simulink model "linear_system_full_state_obs"  (R2021b)
settings: Solver=VariableStepAuto  StartTime=0.0  StopTime=10.0  RelTol=1e-8
undefined symbols (not defined in the file or in its folder): A, B, K
libraries: simulink x2
settings Model: Creator=viking  LastModifiedBy=viking
settings DebuggingCC: UnconnectedInputMsg=none  UnconnectedOutputMsg=none  UnconnectedLineMsg=none
settings ModelReferenceCC: EnableRefExpFcnMdlSchedulingChecks=off
settings RTWCC: DLArmComputeVersion=20.02.1

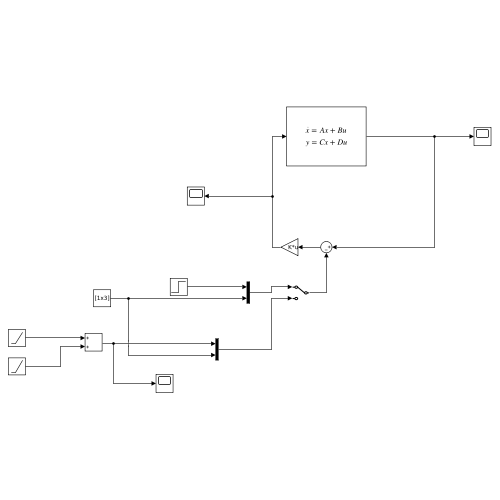
[thumbnail: Simulink's stored preview of the top-level diagram]
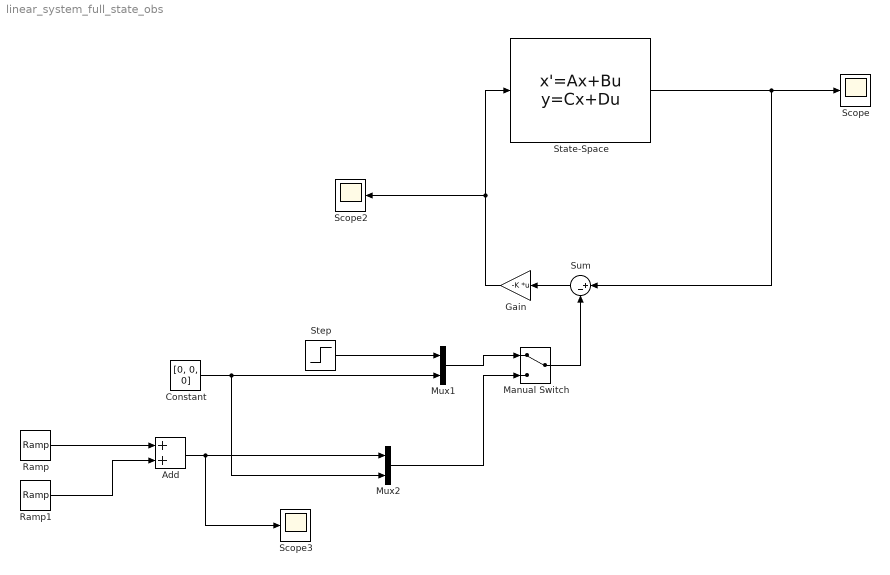
== system linear_system_full_state_obs ==
  Add : Sum
  Constant : Constant  Value=[0, 0, 0]
  Gain : Gain  Gain=-K  Multiplication=Matrix(K*u)
  Manual Switch : ManualSwitch
  Mux1 : Mux  Inputs=2
  Mux2 : Mux  Inputs=2
  Ramp : simulink/Sources/Ramp  slope=1  start=0  InitialOutput=0
  Ramp1 : simulink/Sources/Ramp  slope=-1  start=1  InitialOutput=0
  Scope : Scope
  Scope2 : Scope
  Scope3 : Scope
  State-Space : StateSpace  A=A  B=B  C=eye(4)  D=[0; 0; 0; 0]  InitialCondition=[0, 0, 0, 0]  ContinuousStateAttributes={'theta', 'alpha', 'dtheta', 'dalpha'}
  Step : Step  Time=0.1  SampleTime=0
  Sum : Sum  Inputs=|+-
  wires:
  State-Space/1 -> Sum/1, Scope/1
  Gain/1 -> Scope2/1, State-Space/1
  Sum/1 -> Gain/1
  Step/1 -> Mux1/1
  Manual Switch/1 -> Sum/2
  Mux1/1 -> Manual Switch/1
  Constant/1 -> Mux2/2, Mux1/2
  Mux2/1 -> Manual Switch/2
  Ramp/1 -> Add/1
  Ramp1/1 -> Add/2
  Add/1 -> Scope3/1, Mux2/1
